simulink model "regolazionePI_carrelloPendolo_schema"  (R2022a)
settings: Solver=VariableStepAuto  StartTime=0.0  StopTime=30  RelTol=1e-3
values from neighbouring files (symbols this model uses):
  A = [0      1              0               0 ... (first row only)    [regolazionePI_carrelloPendolo.m]
  B = [0      0 ... (first row only)    [regolazionePI_carrelloPendolo.m]
  C = [1 0 0 0 ... (first row only)    [regolazionePI_carrelloPendolo.m]
  D = [0 0; 0 0]    [regolazionePI_carrelloPendolo.m]
  F = [A-G0*C+B*K P-G0*Q+B*(L); -G1*C S-G1*Q]    [regolazionePI_carrelloPendolo.m]
  G = G'    [regolazionePI_carrelloPendolo.m]
  H = [K L]    [regolazionePI_carrelloPendolo.m]
  Q = [Q eye(r-1)]    [regolazionePI_carrelloPendolo.m]
  S = blkdiag(S, 0)    [regolazionePI_carrelloPendolo.m]
undefined symbols (not defined in the file or in its folder): a1, a2, Angolo_r
settings Model: Creator=Paolo  LastModifiedBy=Paolo

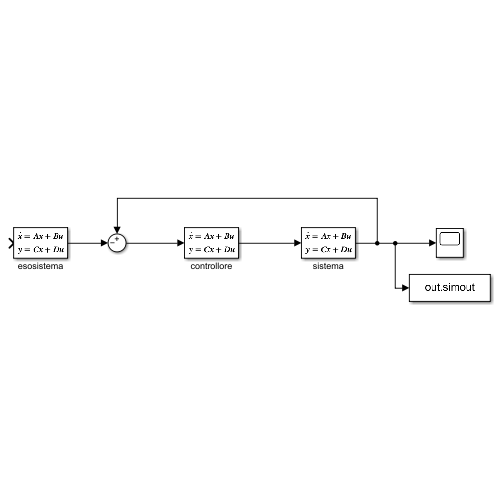
[thumbnail: Simulink's stored preview of the top-level diagram]
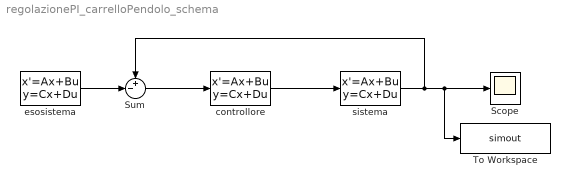
== system regolazionePI_carrelloPendolo_schema ==
  Scope : Scope
  Sum : Sum  Inputs=+-|
  To Workspace : ToWorkspace  VariableName=simout  SaveFormat=Timeseries  SampleTime=-1
  controllore : StateSpace  A=F  B=G  C=H  D=zeros(size(H,1),size(G,2))  InitialCondition=0
  esosistema : StateSpace  A=S  B=zeros(size(S,1))  C=Q  D=zeros(size(Q,1),size(S,1))  InitialCondition=[a1 a2 Angolo_r]
  sistema : StateSpace  A=A  B=B  C=C  D=D  InitialCondition=[1 0 1 0]
  wires:
  controllore/1 -> sistema/1
  esosistema/1 -> Sum/2
  sistema/1 -> To Workspace/1, Scope/1, Sum/1
  Sum/1 -> controllore/1
